simulink model "RailP_DD"  (R2016b)
settings: configuration reference "CodeGenConfigSet" (kept outside this file)
values from neighbouring files (symbols this model uses):
  RailP_pLin_CUR = Calibration.Parameter    [init_RailP_DD.m]
  RailP_pLin_CURX = Calibration.Parameter    [init_RailP_DD.m]
  RailP_tiSRCMaxDefDeb_C = Calibration.Parameter    [init_RailP_DD.m]
  RailP_tiSRCMaxOKDeb_C = Calibration.Parameter    [init_RailP_DD.m]
  RailP_tiSRCMinDefDeb_C = Calibration.Parameter    [init_RailP_DD.m]
  RailP_tiSRCMinOKDeb_C = Calibration.Parameter    [init_RailP_DD.m]
  RailP_uSRCMax_C = Calibration.Parameter    [init_RailP_DD.m]
  RailP_uSRCMin_C = Calibration.Parameter    [init_RailP_DD.m]
undefined symbols (not defined in the file or in its folder): RailP_DD_DT
libraries: CXLib x6
settings Model: Creator=Administrator  LastModifiedBy=zhoutinglin
settings ConfigSetRef: SourceLocation=Base Workspace

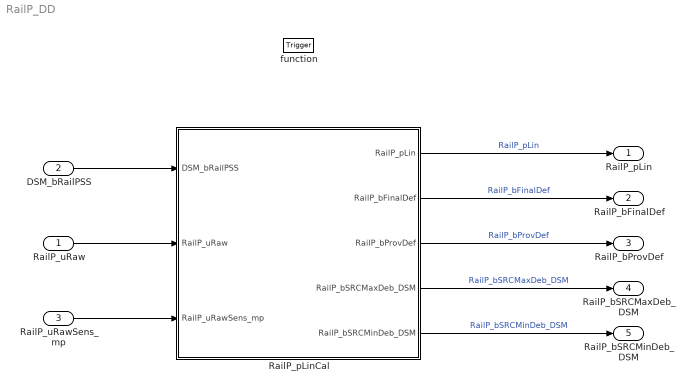
== system RailP_DD ==
  RailP_uRaw : Inport  Tag=mv  Description=Raw value of rail pressure  OutMin=0  OutMax=5000  OutDataTypeStr=Ad_mv
  DSM_bRailPSS : Inport  Description=Status of FId_RailPSS  Port=2  OutMin=0  OutMax=1  OutDataTypeStr=boolean
  RailP_uRawSens_mp : Inport  Tag=mv  Description=Raw value of rail pressure before Peak Selection  Port=3  OutMin=0  OutMax=5000  OutDataTypeStr=Ad_mv
  function : TriggerPort  TriggerType=function-call  VariantControl=Variant
  RailP_pLinCal : Subsystem
  RailP_pLin : Outport  Tag=bar  Description=Fuel pressure  OutMin=0  OutMax=2500  OutDataTypeStr=RailPressure_bar
  RailP_bFinalDef : Outport  Description=Status of final default  Port=2  OutMin=0  OutMax=1  OutDataTypeStr=boolean
  RailP_bProvDef : Outport  Description=Status of provisional default  Port=3  OutMin=0  OutMax=1  OutDataTypeStr=boolean
  RailP_bSRCMaxDeb_DSM : Outport  Description=The debounce result of SRC  Port=4  OutMin=0  OutMax=1  OutDataTypeStr=boolean
  RailP_bSRCMinDeb_DSM : Outport  Description=The debounce result of SRC  Port=5  OutMin=0  OutMax=1  OutDataTypeStr=boolean
  wires:
  RailP_uRaw/1 -> RailP_pLinCal/2(RailP_uRaw)
  DSM_bRailPSS/1 -> RailP_pLinCal/1(DSM_bRailPSS)
  RailP_pLinCal/1(RailP_pLin) -> RailP_pLin/1  "RailP_pLin"
  RailP_pLinCal/2(RailP_bFinalDef) -> RailP_bFinalDef/1  "RailP_bFinalDef"
  RailP_pLinCal/3(RailP_bProvDef) -> RailP_bProvDef/1  "RailP_bProvDef"
  RailP_pLinCal/4(RailP_bSRCMaxDeb_DSM) -> RailP_bSRCMaxDeb_DSM/1  "RailP_bSRCMaxDeb_DSM"
  RailP_pLinCal/5(RailP_bSRCMinDeb_DSM) -> RailP_bSRCMinDeb_DSM/1  "RailP_bSRCMinDeb_DSM"
  RailP_uRawSens_mp/1 -> RailP_pLinCal/3(RailP_uRawSens_mp)

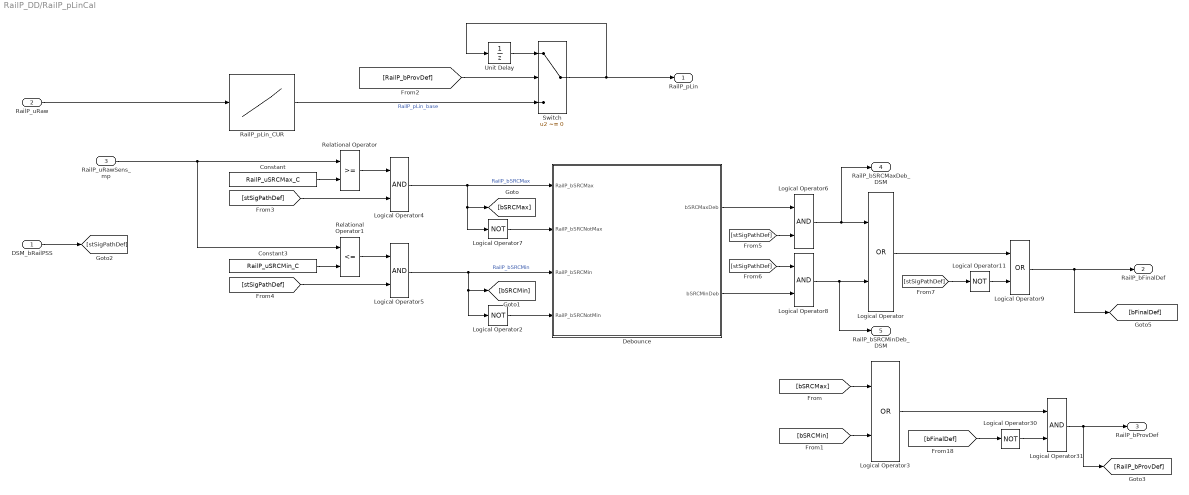
== system RailP_DD/RailP_pLinCal ==
  DSM_bRailPSS : Inport  Description=status of FId_RailPSS  OutMin=0  OutMax=1  OutDataTypeStr=boolean
  RailP_uRaw : Inport  Tag=mv  Description=Raw value of rail pressure  Port=2
  RailP_uRawSens_mp : Inport  Tag=mv  Description=Raw value of rail pressure  Port=3
  Constant : Constant  Value=RailP_uSRCMax_C
  Constant3 : Constant  Value=RailP_uSRCMin_C
  Debounce : Subsystem
  Logical Operator : Logic  Operator=OR  AllPortsSameDT=off  OutDataTypeStr=boolean
  Logical Operator{2,7,11,30} (4 alike) : Logic  Operator=NOT  AllPortsSameDT=off  OutDataTypeStr=boolean
  Logical Operator3 : Logic  Operator=OR  AllPortsSameDT=off  OutDataTypeStr=boolean
  Logical Operator{4..6,8,31} (5 alike) : Logic  AllPortsSameDT=off  OutDataTypeStr=boolean
  Logical Operator9 : Logic  Operator=OR  AllPortsSameDT=off  OutDataTypeStr=boolean
  RailP_pLin_CUR : Lookup_n-D  NumberOfTableDimensions=1  BreakpointsForDimension1=RailP_pLin_CURX  IndexSearchMethod=Linear search  BeginIndexSearchUsingPreviousIndexResult=on  UseOneInputPortForAllInputData=on  Table=RailP_pLin_CUR  ExtrapMethod=Clip  UseLastTableValue=on  InternalRulePriority=Speed  OutDataTypeStr=Inherit: Inherit via back propagation  SaturateOnIntegerOverflow=on
  Relational Operator : RelationalOperator  OutDataTypeStr=boolean  RndMeth=Nearest  InputSameDT=on
  Relational Operator1 : RelationalOperator  Operator=<=  OutDataTypeStr=boolean  RndMeth=Nearest  InputSameDT=on
  Switch : Switch  Criteria=u2 ~= 0
  Unit Delay : UnitDelay  SampleTime=-1
  RailP_pLin : Outport  Tag=bar  Description=Fuel pressure  OutMin=0  OutMax=2500  OutDataTypeStr=RailPressure_bar
  RailP_bFinalDef : Outport  Port=2  OutMin=0  OutMax=1  OutDataTypeStr=boolean
  RailP_bProvDef : Outport  Port=3  OutMin=0  OutMax=1  OutDataTypeStr=boolean
  RailP_bSRCMaxDeb_DSM : Outport  Port=4  OutMin=0  OutMax=1  OutDataTypeStr=boolean
  RailP_bSRCMinDeb_DSM : Outport  Port=5  OutMin=0  OutMax=1  OutDataTypeStr=boolean
  wires:
  Debounce/2(bSRCMinDeb) -> Logical Operator8/2
  Logical Operator9/1 -> [bFinalDef], RailP_bFinalDef/1
  RailP_uRaw/1 -> RailP_pLin_CUR/1
  Logical Operator31/1 -> [RailP_bProvDef], RailP_bProvDef/1
  [bFinalDef] -> Logical Operator30/1
  Relational Operator/1 -> Logical Operator4/1
  Logical Operator7/1 -> Debounce/2(RailP_bSRCNotMax)
  Logical Operator11/1 -> Logical Operator9/2
  DSM_bRailPSS/1 -> [stSigPathDef]
  [stSigPathDef] -> Logical Operator8/1
  Debounce/1(bSRCMaxDeb) -> Logical Operator6/1
  Logical Operator30/1 -> Logical Operator31/2
  Logical Operator3/1 -> Logical Operator31/1
  Relational Operator1/1 -> Logical Operator5/1
  Logical Operator2/1 -> Debounce/4(RailP_bSRCNotMin)
  [stSigPathDef] -> Logical Operator4/2
  Logical Operator4/1 -> Logical Operator7/1, [bSRCMax], Debounce/1(RailP_bSRCMax)  "RailP_bSRCMax"
  [bSRCMax] -> Logical Operator3/1
  Constant/1 -> Relational Operator/2
  Constant3/1 -> Relational Operator1/2
  [stSigPathDef] -> Logical Operator5/2
  [bSRCMin] -> Logical Operator3/2
  [stSigPathDef] -> Logical Operator6/2
  Logical Operator8/1 -> RailP_bSRCMinDeb_DSM/1, Logical Operator/2
  Logical Operator/1 -> Logical Operator9/1
  Logical Operator5/1 -> Logical Operator2/1, [bSRCMin], Debounce/3(RailP_bSRCMin)  "RailP_bSRCMin"
  [stSigPathDef] -> Logical Operator11/1
  Logical Operator6/1 -> RailP_bSRCMaxDeb_DSM/1, Logical Operator/1
  [RailP_bProvDef] -> Switch/2
  RailP_pLin_CUR/1 -> Switch/3  "RailP_pLin_base"
  Switch/1 -> Unit Delay/1, RailP_pLin/1
  Unit Delay/1 -> Switch/1
  RailP_uRawSens_mp/1 -> Relational Operator1/1, Relational Operator/1

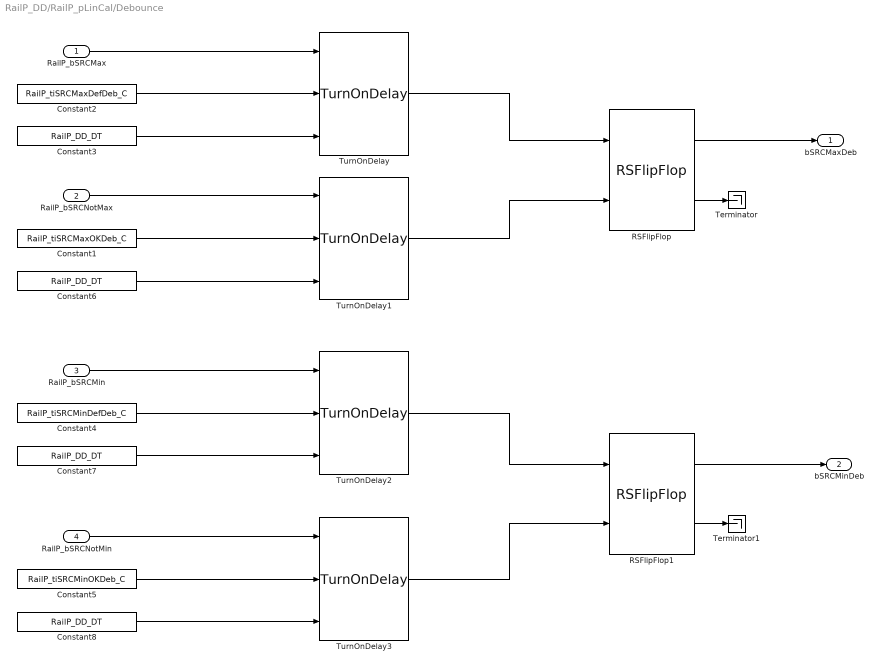
== system RailP_DD/RailP_pLinCal/Debounce ==
  RailP_bSRCMax : Inport
  RailP_bSRCNotMax : Inport  Port=2
  RailP_bSRCMin : Inport  Port=3
  RailP_bSRCNotMin : Inport  Port=4
  Constant1 : Constant  Value=RailP_tiSRCMaxOKDeb_C
  Constant2 : Constant  Value=RailP_tiSRCMaxDefDeb_C
  Constant{3,6..8} (4 alike) : Constant  Value=RailP_DD_DT  OutDataTypeStr=Inherit: Inherit via back propagation
  Constant4 : Constant  Value=RailP_tiSRCMinDefDeb_C
  Constant5 : Constant  Value=RailP_tiSRCMinOKDeb_C
  RSFlipFlop : CXLib/RSFlipFlop
  RSFlipFlop1 : CXLib/RSFlipFlop
  Terminator : Terminator
  Terminator1 : Terminator
  TurnOnDelay{,1..3} (4 alike) : CXLib/TurnOnDelay
  bSRCMaxDeb : Outport
  bSRCMinDeb : Outport  Port=2
  wires:
  Constant8/1 -> TurnOnDelay3/3
  Constant7/1 -> TurnOnDelay2/3
  Constant6/1 -> TurnOnDelay1/3
  Constant3/1 -> TurnOnDelay/3
  RailP_bSRCMax/1 -> TurnOnDelay/1
  RSFlipFlop1/2 -> Terminator1/1
  RSFlipFlop/2 -> Terminator/1
  Constant5/1 -> TurnOnDelay3/2
  TurnOnDelay3/1 -> RSFlipFlop1/2
  RailP_bSRCNotMin/1 -> TurnOnDelay3/1
  TurnOnDelay2/1 -> RSFlipFlop1/1
  RailP_bSRCMin/1 -> TurnOnDelay2/1
  RailP_bSRCNotMax/1 -> TurnOnDelay1/1
  TurnOnDelay/1 -> RSFlipFlop/1
  Constant2/1 -> TurnOnDelay/2
  Constant1/1 -> TurnOnDelay1/2
  Constant4/1 -> TurnOnDelay2/2
  TurnOnDelay1/1 -> RSFlipFlop/2
  RSFlipFlop/1 -> bSRCMaxDeb/1
  RSFlipFlop1/1 -> bSRCMinDeb/1
